simulink model "KiBaM"  (R2017b)
settings: Solver=VariableStepAuto  StartTime=0.0  StopTime=200  RelTol=1e-3
settings Model: Creator=barbot  LastModifiedBy=barbot

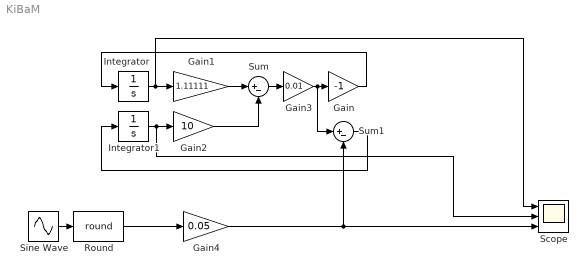
== system KiBaM ==
  Gain : Gain  Gain=-1
  Gain1 : Gain  Gain=1.11111
  Gain2 : Gain  Gain=10
  Gain3 : Gain  Gain=0.01
  Gain4 : Gain  Gain=0.05
  Integrator : Integrator  InitialCondition=9
  Integrator1 : Integrator  InitialCondition=1
  Round : Rounding  Operator=round
  Scope : Scope  NumInputPorts=3
  Sine Wave : Sin  Amplitude=0.5  Bias=0.5  Frequency=0.2  Phase=-1.57  SampleTime=0
  Sum : Sum  Inputs=|+-
  Sum1 : Sum  Inputs=|+-
  wires:
  Sum/1 -> Gain3/1
  Gain1/1 -> Sum/1
  Gain2/1 -> Sum/2
  Gain/1 -> Integrator/1
  Gain3/1 -> Sum1/1, Gain/1
  Sine Wave/1 -> Round/1
  Round/1 -> Gain4/1
  Sum1/1 -> Integrator1/1
  Gain4/1 -> Sum1/2, Scope/3
  Integrator/1 -> Scope/1, Gain1/1
  Integrator1/1 -> Scope/2, Gain2/1
